simulink model "bluetoothLowEnergyWriter"  (R2021a)
settings: Solver=VariableStepAuto  StartTime=0.0  StopTime=2  RelTol=1e-3
undefined symbols (not defined in the file): Fs, ip, usb
libraries: plutoradiolib x1, commsink2 x1, dspsigops x1
settings Model: Creator=Marcin  LastModifiedBy=Marcin

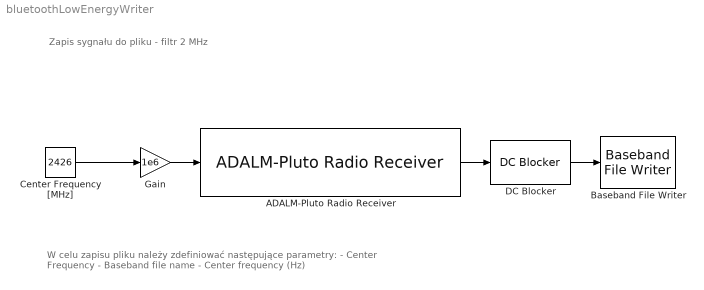
== system bluetoothLowEnergyWriter ==
  note: Zapis sygnału do pliku - filtr 2 MHz
  note: W celu zapisu pliku należy zdefiniować następujące parametry:
      | - Center Frequency
      | - Baseband file name
      | - Center frequency (Hz)
  ADALM-Pluto Radio Receiver : plutoradiolib/ADALM-Pluto Radio Receiver  RadioID=usb:0  uri=ip:10.0.0.200  CenterFrequencySource=Input Port  CenterFrequency=2.4e9  GainSource=AGC Slow Attack  GainSourceBlock=Dialog  Gain=10  ChannelMapping=1  BasebandSampleRate=3000000  OutputDataType=double  SamplesPerFrame=20000  OverflowOutputPort=off  EnableBurstMode=off  NumFramesInBurst=1  ShowAdvancedProperties=off  UseCustomFilter=on  filtPathRates=[983040000 491520000 245760000 122880000 61440000 30720000]  filtCoefficients=[-16 29 24 76 43 19 -52 -59 -29 56 92 55 -56 -129 -96 48 171 153 -28 -215 -228 -10 258 321 72 -295 -435 -162 322 570 290 -330 -727 -464 310 909 699 -249 -1117 -1018 126 1361 1460 97 -1654 -2104 -496 2036 3142 1254 -2666 -5278 -3140 4472 14428 21421 21421 14428 4472 -3140 -5278 -2666 1254 3142 2036 -496 -2104 -1654 97 1460 1361 126 -1018 -1117 -249 699 909 310 -464 -727 -330 290 570 322 -162 -435 -295 72 321 258 -10 -228 -215 -28 153 171 48 -96 -129 -56 55 92 56 -29 -59 -52 19 43 76 24 29 -16]  filtCoefficientSize=112  filtDecimInterpFactor=2  filtGain=-6  filtRFBandwidth=19365514  filterConfigStruct="struct('Rdata',[30720000],'Fpass',[9000000],'Fstop',[11000000],'caldiv',[9],'FIR',[2],'HB1',[2],'PLL_mult',[2],'Apass',[0.1],'Astop',[80],'phEQ',[-1],'HB2',[2],'HB3',[2],'Type','Lowpass','RxTx','Rx','RFbw',[17213779],'DAC_div',[1],'converter_rate',[491520000],'PLL_rate',[983040000],'Fcenter',[0],'wnom',[12049600],'FIRdBmin',[0],'dBstop_FIR',[0],'int_FIR',[1],'FPGAfilter',[0],'firtaps',[-15.703484      28.9472077       23.936501      76.1966891      43.2743274      19.1419701     -52.1877577     -59.2040167     -28.7060831      55.8998818      91.5435001       55.118621     -56.0411108     -129.390896     -96.1904494      48.1112055      171.339703      153.130894     -27.6264314     -215.337621     -227.736712     -10.4711491      258.043362      321.264465      71.5503477     -295.303954     -434.974639     -161.982229      321.606992      569.998332      289.520218     -329.635013     -727.311694     -463.997123      309.897318      908.630232      699.475764      -248.93363      -1117.3688     -1018.21948      125.661596      1360.65503      1459.77593      97.2345126     -1654.00421     -2103.86214     -496.156725      2036.09976      3141.53111      1254.08851      -2665.5149     -5278.27181     -3140.21873      4472.14296       14428.487      21421.1121      21421.1121       14428.487      4472.14296     -3140.21873     -5278.27181      -2665.5149      1254.08851      3141.53111      2036.09976     -496.156725     -2103.86214     -1654.00421      97.2345126      1459.77593      1360.65503      125.661596     -1018.21948      -1117.3688      -248.93363      699.475764      908.630232      309.897318     -463.997123     -727.311694     -329.635013      289.520218      569.998332      321.606992     -161.982229     -434.974639     -295.303954      71.5503477      321.264465      258.043362     -10.4711491     -227.736712     -215.337621     -27.6264314      153.130894      171.339703      48.1112055     -96.1904494     -129.390896     -56.0411108       55.118621      91.5435001      55.8998818     -28.7060831     -59.2040167     -52.1877577      19.1419701      43.2743274      76.1966891       23.936501      28.9472077      -15.703484               0               0               0               0               0               0               0               0               0               0               0               0               0               0               0               0],'nfirtaps',[112],'gain',[-6],'enables','2221','Apass_actual',[0.062571],'Astop_actual',[83.836],'delay',[1.0865e-07],'grpdelayvar',[8.2729e-09],'a1',[1      135196195.8525],'b1',[0      135196195.8525],'a2',[1      151419739.3547823   1.14639687331351e+16  4.339677893856724e+23],'b2',[0                      0                      0  4.339677893856726e+23])"  EnableQuadratureCorrection=on  EnableRFDCCorrection=on  EnableBasebandDCCorrection=on  FrequencyCorrection=0  OverrideSampleTime=off  SampleTime=0.02  DataTimeout=Inf  ENSMPinControlMode=None  BISTLoopbackMode=Disabled  BISTToneInject=Disabled  BISTSignalGen=PRBS  BISTToneFreq=Fs/32  BISTToneLevel=0
      settings: SourceProductBaseCode=PLUTO
  Baseband File Writer : commsink2/Baseband File Writer  Filename=untitled.bb  CenterFrequency=2402e6  Metadata=struct()  NumSamplesToWrite=inf  SimulateUsing=Code generation
      settings: SourceProductBaseCode=CM
  Center Frequency [MHz] : Constant  Value=2426
  DC Blocker : dspsigops/DC Blocker  Algorithm=Subtract mean  NormalizedBandwidth=0.001  Length=8  Order=6  SimulateUsing=Code generation
      settings: SourceProductBaseCode=DS
  Gain : Gain  Gain=1e6
  wires:
  ADALM-Pluto Radio Receiver/1 -> DC Blocker/1
  Gain/1 -> ADALM-Pluto Radio Receiver/1
  Center Frequency [MHz]/1 -> Gain/1
  DC Blocker/1 -> Baseband File Writer/1
